simulink model "CRDI_HPP"  (R2019a)
settings: Solver=FixedStepDiscrete  StartTime=0.0  StopTime=10.0  FixedStep=1  RelTol=1e-3
settings Model: DataDictionary=HPP.sldd  Creator=ADVAIT ELECTRICALS  LastModifiedBy=ADVAIT ELECTRICALS

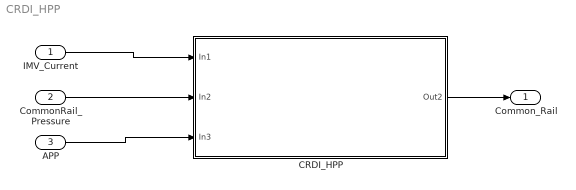
== system CRDI_HPP ==
  IMV_Current : Inport
  CommonRail_Pressure : Inport  Port=2
  APP : Inport  Port=3
  CRDI_HPP : Subsystem
  Common_Rail : Outport
  wires:
  IMV_Current/1 -> CRDI_HPP/1(In1)
  CommonRail_Pressure/1 -> CRDI_HPP/2(In2)
  CRDI_HPP/1(Out2) -> Common_Rail/1
  APP/1 -> CRDI_HPP/3(In3)

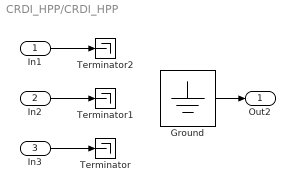
== system CRDI_HPP/CRDI_HPP ==
  In1 : Inport
  In2 : Inport  Port=2
  In3 : Inport  Port=3
  Ground : Ground
  Terminator : Terminator
  Terminator1 : Terminator
  Terminator2 : Terminator
  Out2 : Outport
  wires:
  In3/1 -> Terminator/1
  Ground/1 -> Out2/1
  In2/1 -> Terminator1/1
  In1/1 -> Terminator2/1
